simulink model "alt_dspbuilder_internal_WriteFIFO"  (Simulink 6.3)
settings: Solver=ode45  StartTime=0.0  StopTime=10.0  RelTol=1e-3
InitFcn:
  | %% DSPBuilder Start
  | alt_dspbuilder_update_model(bdroot)
  | %% DSPBuilder End
libraries: allblocks_alteradspbuilder2 x9
settings Model: Creator=cpurcell  LastModifiedBy=cpurcell
settings DebuggingCC: AlgebraicLoopMsg=none  MultiTaskCondExecSysMsg=none  StrictBusMsg=Warning
settings RTWCC: IncludeERTFirstTime=on
settings CodeAppCC: CustomSymbolStrType=$N$R$M

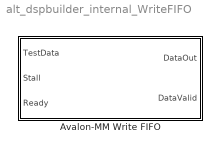
== system alt_dspbuilder_internal_WriteFIFO ==
  Avalon-MM Write FIFO : Subsystem  mask(Avalon-MM Write FIFO AlteraBlockSet){sgn=Unsigned Integer, bwl=8, bwr=0, depth=16, burst=8}
      mask prompts: sgn "Data Type"; bwl "[number of bits].[]"; bwr "[].[number of bits]"; depth "FIFO Depth"; burst "Maximum Burst Size"
      mask help:
      | Avalon-MM Write FIFO
      |
      | Implements a FIFO with Avalon-MM connectivity. Used to receive data from other Avalon-MM peripheralswhen connected in SOPC Builder.
      |
      | Inputs:
      | TestData - Connect to Simulink blocks.
      | 	Used to provide simulation data to the Avalon-MM Write FIFO.
      | Stall - Connect to Simulink blocks.
      | 	Used to simulate stall conditions of the Avalon-MM bus.
      | Ready - Connect to DSP Builder blocks.
      | 	Used to indicate that the downstream hardware is ready for data.
      |
      | Outputs:
      | DataOut - Connect to DSP Builder blocks.
      | 	Corresponds to the oldest unsent data sample received on the TestData port.
      | DataValid - Connect to DSP Builder blocks.
      | 	Asserted whenever DataOut corresponds to real data.
      mask init:
      | alt_dspbuilder_internal_AvalonFIFO_Init(gcb,0,1, bwl,bwr,depth,burst);
      settings: CopyFcn=set_param(gcbh,'LinkStatus','none');
      mask Help: helpview(fullfile(alt_dspbuilder_get_quartus_rootdir, 'dsp_builder', 'docs', 'AvalonWriteFifo.html'))
      mask StyleString: popup(Signed Integer|Signed Fractional|Unsigned Integer),edit,edit,edit,edit
      mask CallbackString: alt_dspbuilder_internal_AvalonFIFO_Init(gcb,0,0);||||

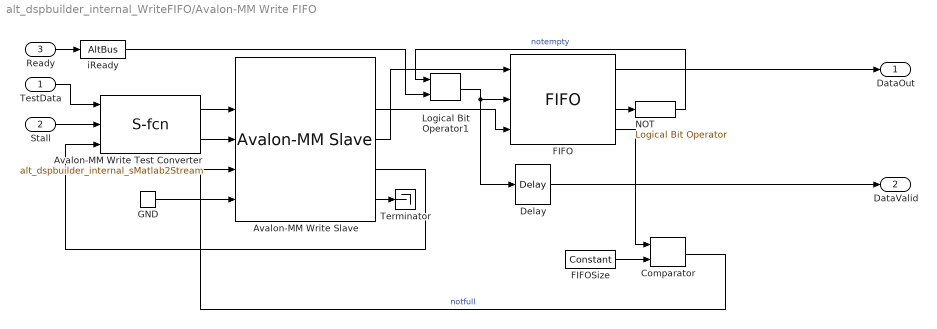
== system alt_dspbuilder_internal_WriteFIFO/Avalon-MM Write FIFO ==
  TestData : Inport
  Stall : Inport  Port=2
  Ready : Inport  Port=3
  Avalon-MM Write Slave : allblocks_alteradspbuilder2/Avalon-MM Slave  iofile=C:\DOCUME~1\cpurcell\LOCALS~1\Temp\tb_tp303539\tp303539_Avalon-MM+Write+FIFO_Avalon-MM+Write+Slave_address.salt,C:\DOCUME~1\cpurcell\LOCALS~1\Temp\tb_tp303539\tp303539_Avalon-MM+Write+FIFO_Avalon-MM+Write+Slave_write.salt,C:\DOCUME~1\cpurcell\LOCALS~1\Temp\tb_tp303539\tp303539_Avalon-MM+Write+FIFO_Avalon-MM+Write+Slave_writedata.salt,C:\DOCUME~1\cpurcell\LOCALS~1\Temp\tb_tp303539\tp303539_Avalon-MM+Write+FIFO_Avalon-MM+Write+Slave_readyfordata.capture,C:\DOCUME~1\cpurcell\LOCALS~1\Temp\tb_tp303539\tp303539_Avalon-MM+Write+FIFO_Avalon-MM+Write+Slave_endofpacket.capture,  SpecifyClock=off  clock=clock  addrWidth=2  addrAlignment=Dynamic  addrType=Write  BusType=Unsigned Integer  bwl=bwl  bwr=bwr  byteEnable=off  flowCtrl=on  pipeline=off  waitStateFormat=Fixed  readWaitStateCycles=0  writeWaitStateCycles=0  readLatencyFormat=Fixed  readLatencyCycles=0  burst=off  maxBurst=burst  irq=off  receiveBeginTransfer=off  useChipSelect=off  PORTTYPE=Output
  Avalon-MM Write Test Converter : S-Function  FunctionName=alt_dspbuilder_internal_sMatlab2Stream  Parameters=-1 1000000
      mask Display:
      | port_label('input', 1, 'TestData');
      | port_label('input', 2, 'Stall');
      | port_label('input', 3, 'Ready');
      | port_label('output', 1, 'Write');
      | port_label('output', 2, 'WriteData');
  Comparator : allblocks_alteradspbuilder2/Comparator  direction=a < b
  Delay : allblocks_alteradspbuilder2/Delay  pipeline=1  ClockPhase=1  use_ena=off  use_sclr=off
  FIFO : allblocks_alteradspbuilder2/FIFO  numwords=depth  BusType=Unsigned Integer  bwl=bwl  bwr=bwr  ram_type=AUTO  use_sclr=off  use_les_only=off  showahead_mode=off
  FIFOSize : allblocks_alteradspbuilder2/Constant  mask_cst=depth -2  BusType=Unsigned Integer  bwl=ceil(log2(depth-1))  bwr=0  SpecifyClock=off
  GND : allblocks_alteradspbuilder2/GND  SpecifyClock=off
  Logical Bit Operator1 : allblocks_alteradspbuilder2/Logical Bit Operator  LogicalOperator=AND  user_inputs=2
  NOT : allblocks_alteradspbuilder2/Logical Bit Operator  LogicalOperator=NOT  user_inputs=2
  Terminator : Terminator
  iReady : allblocks_alteradspbuilder2/AltBus  BusType=Single Bit  bwl=1  bwr=0  saturate=off
  DataOut : Outport
  DataValid : Outport  Port=2
  wires:
  Ready/1 -> iReady/1
  Avalon-MM Write Slave/3 -> FIFO/1
  Avalon-MM Write Slave/2 -> FIFO/3
  FIFO/3 -> NOT/1
  FIFO/1 -> DataOut/1
  Avalon-MM Write Test Converter/1 -> Avalon-MM Write Slave/2
  Avalon-MM Write Slave/4 -> Avalon-MM Write Test Converter/3
  TestData/1 -> Avalon-MM Write Test Converter/1
  GND/1 -> Avalon-MM Write Slave/5
  NOT/1 -> Logical Bit Operator1/1  "notempty"
  iReady/1 -> Logical Bit Operator1/2
  Delay/1 -> DataValid/1
  Avalon-MM Write Test Converter/2 -> Avalon-MM Write Slave/3
  Stall/1 -> Avalon-MM Write Test Converter/2
  Avalon-MM Write Slave/5 -> Terminator/1
  Comparator/1 -> Avalon-MM Write Slave/4  "notfull"
  FIFOSize/1 -> Comparator/2
  FIFO/4 -> Comparator/1
  Logical Bit Operator1/1 -> FIFO/2, Delay/1
